simulink model "Auto_Identification_2degre"  (R2015a)
settings: Solver=ode3  StartTime=0.0  StopTime=10  FixedStep=0.01  RelTol=1e-3
PostLoadFcn:
  | load('LeftOutput_Measures.mat');
  | load('LeftOutput_Measures.mat');
  | Parametres_Rover
undefined symbols (not defined in the file): KL2, TdL2, TwL, ZetaL
settings Model: Creator=tbaroche  LastModifiedBy=tbaroche

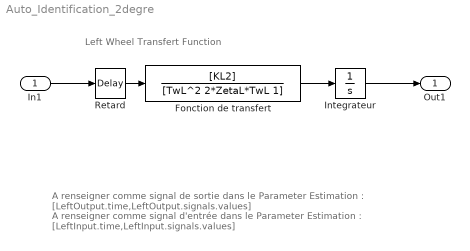
== system Auto_Identification_2degre ==
  note: Left Wheel Transfert Function
  note: A renseigner comme signal d'entrée dans le Parameter Estimation : [LeftInput.time,LeftInput.signals.values]
  note: A renseigner comme signal de sortie dans le Parameter Estimation : [LeftOutput.time,LeftOutput.signals.values]
  In1 : Inport
  Fonction de transfert : TransferFcn  Numerator=[KL2]  Denominator=[TwL^2 2*ZetaL*TwL 1]
  Integrateur : Integrator
  Retard : TransportDelay  DelayTime=TdL2
  Out1 : Outport
  wires:
  Integrateur/1 -> Out1/1
  Retard/1 -> Fonction de transfert/1
  In1/1 -> Retard/1
  Fonction de transfert/1 -> Integrateur/1
